simulink subsystem "Tractive_Motor_Ring_Four_Motors_subsysref"  (R2020a)
settings: Solver=VariableStepAuto  StartTime=0.0  StopTime=10.0  RelTol=1e-3
undefined symbols (not defined in the file): RING_STATUS
settings Model: Creator=Kiera  LastModifiedBy=Kiera

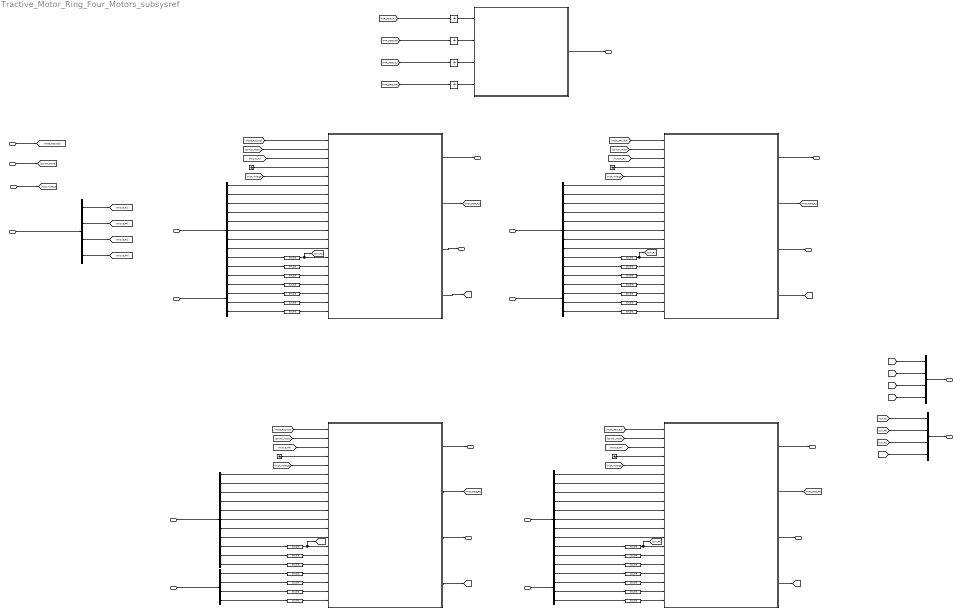
== system Tractive_Motor_Ring_Four_Motors_subsysref ==
  MSR_Mode_Request : Inport  OutDataTypeStr=Enum: MSR_REQUEST
  Control_Mode : Inport  Port=2
  Accumulator_Voltage : Inport  Port=3
  Torque_Requests : Inport  Port=4  OutDataTypeStr=Bus: TorqueRequests
  Actual_Values1_FL : Inport  Port=5  OutDataTypeStr=Bus: AmkActualValues1
      settings: VarSizeSig=Yes
  Actual_Values1_FR : Inport  Port=6  OutDataTypeStr=Bus: AmkActualValues1
  Actual_Values1_RL : Inport  Port=7  OutDataTypeStr=Bus: AmkActualValues1
  Actual_Values1_RR : Inport  Port=8  OutDataTypeStr=Bus: AmkActualValues1
  Actual_Values2_FL : Inport  Port=9  OutDataTypeStr=Bus: AmkActualValues2
  Actual_Values2_FR : Inport  Port=10  OutDataTypeStr=Bus: AmkActualValues2
  Actual_Values2_RL : Inport  Port=11  OutDataTypeStr=Bus: AmkActualValues2
  Actual_Values2_RR : Inport  Port=12  OutDataTypeStr=Bus: AmkActualValues2
  Bus Creator : BusCreator  Inputs=4  OutDataTypeStr=Bus: TorqueLimits
      settings: InheritFromInputs=off
  Bus Creator1 : BusCreator  Inputs=4  OutDataTypeStr=Bus: MotorRPMs
      settings: InheritFromInputs=off
  Bus Selector : BusSelector  OutputSignals=TorqueFrontLeft,TorqueFrontRight,TorqueRearLeft,TorqueRearRight
  Bus Selector{1,3,5,7} (4 alike) : BusSelector  OutputSignals=AMK_bSystemReady,AMK_bError,AMK_bWarn,AMK_bQuitDcOn,AMK_bDcOn,AMK_bQuitInverterOn,AMK_bInverterOn,AMK_bDerating,AMK_ActualVelocity,AMK_TorqueCurrent,AMK_MagnetizingCurrent
  Bus Selector{2,4,6,8} (4 alike) : BusSelector  OutputSignals=AMK_TempMotor,AMK_TempInverter,AMK_ErrorInfo,AMK_TempIGBT
  Data Type Conversion{1..28} (28 alike) : DataTypeConversion  OutDataTypeStr=double
  Ground{,1..3} (4 alike) : Ground
  MasterTmr : Stateflow chart  TreatAsAtomicUnit=on
  Subsystem Reference{,1..3} (4 alike) : Subsystem  ReferencedSubsystem=Tractive_Motor_Ring_Single_Motor_subsys
  Unit Delay{,1..3} (4 alike) : UnitDelay  InitialCondition=RING_STATUS.OFF  SampleTime=-1  HasFrameUpgradeWarning=on
  AMK_Setpoints_FL : Outport  OutDataTypeStr=Bus: AmkSetpoints  VectorParamsAs1DForOutWhenUnconnected=off
  AMK_Setpoints_FR : Outport  Port=2  OutDataTypeStr=Bus: AmkSetpoints  VectorParamsAs1DForOutWhenUnconnected=off
  AMK_Setpoints_RL : Outport  Port=3  OutDataTypeStr=Bus: AmkSetpoints  VectorParamsAs1DForOutWhenUnconnected=off
  AMK_Setpoints_RR : Outport  Port=4  OutDataTypeStr=Bus: AmkSetpoints  VectorParamsAs1DForOutWhenUnconnected=off
  Torque_Limits : Outport  Port=5  OutDataTypeStr=Bus: TorqueLimits  VectorParamsAs1DForOutWhenUnconnected=off
  TMR_State : Outport  Port=6  VectorParamsAs1DForOutWhenUnconnected=off
  Leaf_state_FL : Outport  Port=7  VectorParamsAs1DForOutWhenUnconnected=off
  Leaf_state_FR : Outport  Port=8  VectorParamsAs1DForOutWhenUnconnected=off
  Leaf_state_RL : Outport  Port=9  VectorParamsAs1DForOutWhenUnconnected=off
  Leaf_state_RR : Outport  Port=10  VectorParamsAs1DForOutWhenUnconnected=off
  MotorRpms : Outport  Port=11  OutDataTypeStr=Bus: MotorRPMs  VectorParamsAs1DForOutWhenUnconnected=off
  wires:
  Subsystem Reference1/1 -> AMK_Setpoints_FL/1
  Bus Selector1/7 -> Subsystem Reference3/12  "<AMK_bInverterOn>"
  Bus Selector3/2 -> Subsystem Reference2/7  "<AMK_bError>"
  [Control_Mode] -> Subsystem Reference1/2
  Bus Selector3/9 -> Data Type Conversion5/1  "<AMK_ActualVelocity>"
  Bus Selector1/3 -> Subsystem Reference3/8  "<AMK_bWarn>"
  Bus Selector2/2 -> Data Type Conversion20/1  "<AMK_TempInverter>"
  Bus Selector3/3 -> Subsystem Reference2/8  "<AMK_bWarn>"
  Bus Selector/4 -> [Torque_RR]  "<TorqueRearRight>"
  Actual_Values2_RL/1 -> Bus Selector8/1
  Bus Selector7/4 -> Subsystem Reference/9  "<AMK_bQuitDcOn>"
  Bus Selector1/6 -> Subsystem Reference3/11  "<AMK_bQuitInverterOn>"
  Bus Selector7/8 -> Subsystem Reference/13  "<AMK_bDerating>"
  Bus Selector7/11 -> Data Type Conversion10/1  "<AMK_MagnetizingCurrent>"
  [High_Voltage] -> Subsystem Reference3/5
  [Mode_Request] -> Subsystem Reference3/1
  Bus Selector1/1 -> Subsystem Reference3/6  "<AMK_bSystemReady>"
  Subsystem Reference1/3 -> Leaf_state_FL/1
  Bus Selector4/1 -> Data Type Conversion22/1  "<AMK_TempMotor>"
  Control_Mode/1 -> [Control_Mode]
  [Torque_RR] -> Subsystem Reference3/3
  [Mode_Request] -> Subsystem Reference2/1
  Bus Selector4/3 -> Data Type Conversion26/1  "<AMK_ErrorInfo>"
  Actual_Values2_FR/1 -> Bus Selector4/1
  Bus Selector1/5 -> Subsystem Reference3/10  "<AMK_bDcOn>"
  Subsystem Reference/3 -> Leaf_state_RL/1
  Subsystem Reference3/4 -> [TL_RR]
  Accumulator_Voltage/1 -> [High_Voltage]
  Actual_Values2_RR/1 -> Bus Selector2/1
  Actual_Values1_FL/1 -> Bus Selector5/1
  Bus Selector3/7 -> Subsystem Reference2/12  "<AMK_bInverterOn>"
  Bus Selector1/10 -> Data Type Conversion6/1  "<AMK_TorqueCurrent>"
  [Control_Mode] -> Subsystem Reference/2
  [High_Voltage] -> Subsystem Reference/5
  Bus Selector7/1 -> Subsystem Reference/6  "<AMK_bSystemReady>"
  Actual_Values2_FL/1 -> Bus Selector6/1
  Subsystem Reference1/4 -> [TL_FL]
  Bus Selector1/2 -> Subsystem Reference3/7  "<AMK_bError>"
  Bus Selector/1 -> [Torque_FL]  "<TorqueFrontLeft>"
  [Mode_Request] -> Subsystem Reference/1
  Bus Selector8/3 -> Data Type Conversion28/1  "<AMK_ErrorInfo>"
  Subsystem Reference1/2 -> [TMR_State_FL]
  [Control_Mode] -> Subsystem Reference3/2
  Bus Selector/2 -> [Torque_FR]  "<TorqueFrontRight>"
  [Mode_Request] -> Subsystem Reference1/1
  Bus Selector5/11 -> Data Type Conversion12/1  "<AMK_MagnetizingCurrent>"
  Bus Selector1/4 -> Subsystem Reference3/9  "<AMK_bQuitDcOn>"
  Bus Selector3/10 -> Data Type Conversion3/1  "<AMK_TorqueCurrent>"
  Bus Selector5/9 -> Data Type Conversion2/1  "<AMK_ActualVelocity>"
  Bus Selector6/4 -> Data Type Conversion15/1  "<AMK_TempIGBT>"
  Bus Selector5/6 -> Subsystem Reference1/11  "<AMK_bQuitInverterOn>"
  Bus Selector3/4 -> Subsystem Reference2/9  "<AMK_bQuitDcOn>"
  Subsystem Reference3/3 -> Leaf_state_RR/1
  Bus Selector8/4 -> Data Type Conversion18/1  "<AMK_TempIGBT>"
  Subsystem Reference2/3 -> Leaf_state_FR/1
  Bus Creator/1 -> Torque_Limits/1
  MSR_Mode_Request/1 -> [Mode_Request]
  Bus Selector5/4 -> Subsystem Reference1/9  "<AMK_bQuitDcOn>"
  Bus Selector8/1 -> Data Type Conversion16/1  "<AMK_TempMotor>"
  [Torque_FR] -> Subsystem Reference2/3
  Bus Selector2/3 -> Data Type Conversion27/1  "<AMK_ErrorInfo>"
  Bus Selector5/5 -> Subsystem Reference1/10  "<AMK_bDcOn>"
  Data Type Conversion6/1 -> Subsystem Reference3/15
  [rpm_RR] -> Bus Creator1/4  "RpmRearRight"
  Data Type Conversion15/1 -> Subsystem Reference1/20
  Subsystem Reference/2 -> [TMR_State_RL]
  Bus Selector7/5 -> Subsystem Reference/10  "<AMK_bDcOn>"
  Data Type Conversion27/1 -> Subsystem Reference3/19
  Unit Delay1/1 -> MasterTmr/2(TmrStatusFr)
  [High_Voltage] -> Subsystem Reference1/5
  [TMR_State_RR] -> Unit Delay3/1  "TmrStatusRr"
  [rpm_FR] -> Bus Creator1/2  "RpmFrontRight"
  [High_Voltage] -> Subsystem Reference2/5
  Bus Selector5/2 -> Subsystem Reference1/7  "<AMK_bError>"
  [TL_RL] -> Bus Creator/3  "TorqueLimitRearLeft"
  Bus Selector3/5 -> Subsystem Reference2/10  "<AMK_bDcOn>"
  Ground3/1 -> Subsystem Reference/4
  Bus Selector6/1 -> Data Type Conversion13/1  "<AMK_TempMotor>"
  Data Type Conversion10/1 -> Subsystem Reference/16
  Data Type Conversion11/1 -> Subsystem Reference/14, [rpm_RL]
  Data Type Conversion4/1 -> Subsystem Reference2/16
  Bus Selector5/3 -> Subsystem Reference1/8  "<AMK_bWarn>"
  Bus Selector2/1 -> Data Type Conversion19/1  "<AMK_TempMotor>"
  Unit Delay/1 -> MasterTmr/1(TmrStatusFl)
  Subsystem Reference/4 -> [TL_RL]
  Subsystem Reference3/2 -> [TMR_State_RR]
  Bus Selector7/7 -> Subsystem Reference/12  "<AMK_bInverterOn>"
  [rpm_FL] -> Bus Creator1/1  "RpmFrontLeft"
  Bus Selector2/4 -> Data Type Conversion21/1  "<AMK_TempIGBT>"
  Data Type Conversion9/1 -> Subsystem Reference/15
  Bus Selector3/11 -> Data Type Conversion4/1  "<AMK_MagnetizingCurrent>"
  Bus Selector7/10 -> Data Type Conversion9/1  "<AMK_TorqueCurrent>"
  Unit Delay3/1 -> MasterTmr/4(TmrStatusRr)
  Data Type Conversion28/1 -> Subsystem Reference/19
  Data Type Conversion7/1 -> Subsystem Reference3/16
  Bus Selector1/9 -> Data Type Conversion8/1  "<AMK_ActualVelocity>"
  Bus Selector7/6 -> Subsystem Reference/11  "<AMK_bQuitInverterOn>"
  Bus Selector1/11 -> Data Type Conversion7/1  "<AMK_MagnetizingCurrent>"
  [rpm_RL] -> Bus Creator1/3  "RpmRearLeft"
  Bus Selector8/2 -> Data Type Conversion17/1  "<AMK_TempInverter>"
  Data Type Conversion5/1 -> Subsystem Reference2/14, [rpm_FR]
  Bus Selector6/3 -> Data Type Conversion25/1  "<AMK_ErrorInfo>"
  Bus Creator1/1 -> MotorRpms/1
  Subsystem Reference2/4 -> [TL_FR]
  Data Type Conversion18/1 -> Subsystem Reference/20
  Bus Selector5/1 -> Subsystem Reference1/6  "<AMK_bSystemReady>"
  Bus Selector/3 -> [Torque_RL]  "<TorqueRearLeft>"
  Data Type Conversion16/1 -> Subsystem Reference/17
  Data Type Conversion26/1 -> Subsystem Reference2/19
  Subsystem Reference2/2 -> [TMR_State_FR]
  [TL_FL] -> Bus Creator/1  "TorqueLimitFrontLeft"
  Data Type Conversion3/1 -> Subsystem Reference2/15
  Bus Selector3/1 -> Subsystem Reference2/6  "<AMK_bSystemReady>"
  Data Type Conversion13/1 -> Subsystem Reference1/17
  Data Type Conversion14/1 -> Subsystem Reference1/18
  Data Type Conversion17/1 -> Subsystem Reference/18
  Bus Selector7/3 -> Subsystem Reference/8  "<AMK_bWarn>"
  Data Type Conversion2/1 -> Subsystem Reference1/14, [rpm_FL]
  Data Type Conversion8/1 -> Subsystem Reference3/14, [rpm_RR]
  Bus Selector5/7 -> Subsystem Reference1/12  "<AMK_bInverterOn>"
  Unit Delay2/1 -> MasterTmr/3(TmrStatusRl)
  Data Type Conversion1/1 -> Subsystem Reference1/15
  Actual_Values1_RR/1 -> Bus Selector1/1
  Data Type Conversion12/1 -> Subsystem Reference1/16
  Bus Selector7/2 -> Subsystem Reference/7  "<AMK_bError>"
  [Torque_RL] -> Subsystem Reference/3
  [TMR_State_RL] -> Unit Delay2/1  "TmrStatusRl"
  [TMR_State_FR] -> Unit Delay1/1  "TmrStatusFr"
  Data Type Conversion24/1 -> Subsystem Reference2/20
  Ground/1 -> Subsystem Reference3/4
  Bus Selector5/10 -> Data Type Conversion1/1  "<AMK_TorqueCurrent>"
  Bus Selector3/8 -> Subsystem Reference2/13  "<AMK_bDerating>"
  MasterTmr/1(TmrState) -> TMR_State/1
  Actual_Values1_RL/1 -> Bus Selector7/1
  Ground2/1 -> Subsystem Reference1/4
  [Control_Mode] -> Subsystem Reference2/2
  Torque_Requests/1 -> Bus Selector/1
  Data Type Conversion19/1 -> Subsystem Reference3/17
  [TL_FR] -> Bus Creator/2  "TorqueLimitFrontRight"
  [TMR_State_FL] -> Unit Delay/1  "TmrStatusFl"
  Data Type Conversion22/1 -> Subsystem Reference2/17
  Data Type Conversion25/1 -> Subsystem Reference1/19
  Bus Selector5/8 -> Subsystem Reference1/13  "<AMK_bDerating>"
  Subsystem Reference3/1 -> AMK_Setpoints_RR/1
  Bus Selector4/2 -> Data Type Conversion23/1  "<AMK_TempInverter>"
  Bus Selector1/8 -> Subsystem Reference3/13  "<AMK_bDerating>"
  Actual_Values1_FR/1 -> Bus Selector3/1
  Data Type Conversion23/1 -> Subsystem Reference2/18
  Bus Selector4/4 -> Data Type Conversion24/1  "<AMK_TempIGBT>"
  [Torque_FL] -> Subsystem Reference1/3
  Subsystem Reference2/1 -> AMK_Setpoints_FR/1
  Data Type Conversion21/1 -> Subsystem Reference3/20
  [TL_RR] -> Bus Creator/4  "TorqueLimitRearRight"
  Bus Selector3/6 -> Subsystem Reference2/11  "<AMK_bQuitInverterOn>"
  Subsystem Reference/1 -> AMK_Setpoints_RL/1
  Data Type Conversion20/1 -> Subsystem Reference3/18
  Ground1/1 -> Subsystem Reference2/4
  Bus Selector6/2 -> Data Type Conversion14/1  "<AMK_TempInverter>"
  Bus Selector7/9 -> Data Type Conversion11/1  "<AMK_ActualVelocity>"

== stateflow chart Tractive_Motor_Ring_Four_Motors_subsysref/MasterTmr ==
  state SHUTDOWN
    entry:
    TmrState = RING_STATUS.SHUTDOWN_COMPLETE_HV;
  state OFF
    entry:
    TmrState = RING_STATUS.OFF;
  state STARTUP_LV
    entry:
    TmrState = RING_STATUS.STARTUP_COMPLETE_LV;
  state RUNNING
    entry:
    TmrState = RING_STATUS.RUNNING;
  state STARTUP_HV1
    entry:
    TmrState = RING_STATUS.STARTUP_COMPLETE_HV;
  (default) -> OFF
  OFF -> STARTUP_LV : [TmrStatusFl == RING_STATUS.STARTUP_COMPLETE_LV && ...
      | TmrStatusFr == RING_STATUS.STARTUP_COMPLETE_LV && ...
      | TmrStatusRl == RING_STATUS.STARTUP_COMPLETE_LV && ...
      | TmrStatusRr == RING_STATUS.STARTUP_COMPLETE_LV]
  RUNNING -> SHUTDOWN : [TmrStatusFl == RING_STATUS.SHUTDOWN_COMPLETE_HV && ...
      | TmrStatusFr == RING_STATUS.SHUTDOWN_COMPLETE_HV && ...
      | TmrStatusRl == RING_STATUS.SHUTDOWN_COMPLETE_HV && ...
      | TmrStatusRr == RING_STATUS.SHUTDOWN_COMPLETE_HV]
  STARTUP_HV1 -> RUNNING : [TmrStatusFl == RING_STATUS.RUNNING && ...
      | TmrStatusFr == RING_STATUS.RUNNING && ...
      | TmrStatusRl == RING_STATUS.RUNNING && ...
      | TmrStatusRr == RING_STATUS.RUNNING]
  STARTUP_LV -> STARTUP_HV1 : [TmrStatusFl == RING_STATUS.STARTUP_COMPLETE_HV && ...
      | TmrStatusFr == RING_STATUS.STARTUP_COMPLETE_HV && ...
      | TmrStatusRl == RING_STATUS.STARTUP_COMPLETE_HV && ...
      | TmrStatusRr == RING_STATUS.STARTUP_COMPLETE_HV]
  data: TmrStatusFl input Enum: RING_STATUS; TmrStatusFr input Enum: RING_STATUS; TmrStatusRl input Enum: RING_STATUS; TmrStatusRr input Enum: RING_STATUS; TmrState output Enum: RING_STATUS =RING_STATUS.OFF
